simulink subsystem "FORCESANDTORQUES"  (R2025b)
settings: Solver=VariableStepAuto  StartTime=0.0  StopTime=10.0  RelTol=1e-3
model mask{refSurf=0, dc=0}
  mask prompts: refSurf "Reference aerodynamic surface [m2]"; dc "Drag coefficient [-]"
libraries: sharedutil x1, aerolibutil x1
settings Model: Creator=antoniohernandez-rodiciomateos  LastModifiedBy=antoniohernandez-rodiciomateos

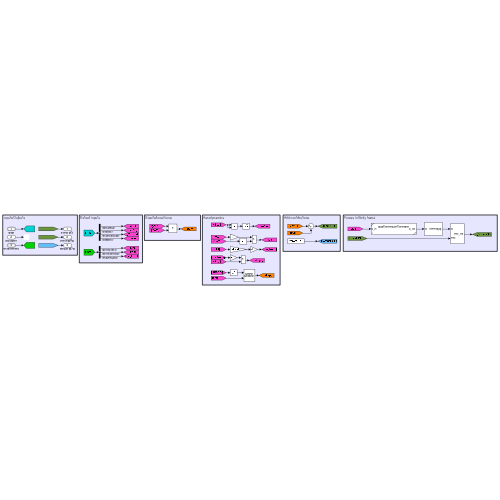
[thumbnail: Simulink's stored preview of the top-level diagram]
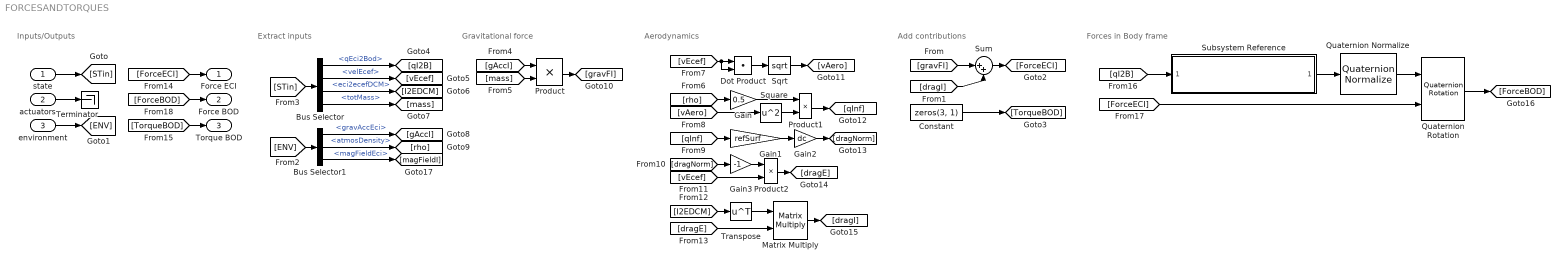
== system FORCESANDTORQUES ==
  note: Inputs/Outputs
  note: Extract inputs
  note: Gravitational force
  note: Aerodynamics
  note: Add contributions
  note: Forces in Body frame
  state : Inport  OutDataTypeStr=Bus: state_bus
  actuators : Inport  Port=2
  environment : Inport  Port=3  OutDataTypeStr=Bus: environment_bus
  Bus Selector : BusSelector  OutputSignals=qEci2Bod,velEcef,eci2ecefDCM,totMass
  Bus Selector1 : BusSelector  OutputSignals=gravAccEci,atmosDensity,magFieldEci
  Constant : Constant  Value=zeros(3, 1)
  Dot Product : DotProduct  OutDataTypeStr=Inherit: Inherit via internal rule
  Gain : Gain  Gain=0.5
  Gain1 : Gain  Gain=refSurf
  Gain2 : Gain  Gain=dc
  Gain3 : Gain  Gain=-1
  Matrix Multiply : Product  Multiplication=Matrix(*)
  Product : Product
  Product1 : Product
  Product2 : Product
  Quaternion Normalize : sharedutil/Quaternion Normalize  aMode=aMode
  Quaternion Rotation : aerolibutil/Quaternion Rotation
  Sqrt : Sqrt
  Square : Math  Operator=square
  Subsystem Reference : Subsystem  ReferencedSubsystem=quatConventionConverter  conversion=q4 to q0
  Sum : Sum  Inputs=|++
  Terminator : Terminator
  Transpose : Math  Operator=transpose
  Force ECI : Outport  OutDataTypeStr=double  PortDimensions=[3 1]
  Force BOD : Outport  Port=2  OutDataTypeStr=double  PortDimensions=[3 1]
  Torque BOD : Outport  Port=3  OutDataTypeStr=double  PortDimensions=[3 1]
  wires:
  actuators/1 -> Terminator/1
  state/1 -> [STin]
  environment/1 -> [ENV]
  [ForceECI] -> Force ECI/1
  [STin] -> Bus Selector/1
  Bus Selector/1 -> [qI2B]  "<qEci2Bod>"
  Bus Selector/2 -> [vEcef]  "<velEcef>"
  Bus Selector/3 -> [I2EDCM]  "<eci2ecefDCM>"
  Bus Selector/4 -> [mass]  "<totMass>"
  [ENV] -> Bus Selector1/1
  Bus Selector1/1 -> [gAccI]  "<gravAccEci>"
  Bus Selector1/2 -> [rho]  "<atmosDensity>"
  [gAccI] -> Product/1
  [mass] -> Product/2
  Product/1 -> [gravFI]
  [vEcef] -> Dot Product/2, Dot Product/1
  Dot Product/1 -> Sqrt/1
  Sqrt/1 -> [vAero]
  [rho] -> Gain/1
  [vAero] -> Square/1
  Gain/1 -> Product1/1
  Square/1 -> Product1/2
  Product1/1 -> [qInf]
  [qInf] -> Gain1/1
  Gain1/1 -> Gain2/1
  Gain2/1 -> [dragNorm]
  [dragNorm] -> Gain3/1
  Gain3/1 -> Product2/1
  [vEcef] -> Product2/2
  Product2/1 -> [dragE]
  [I2EDCM] -> Transpose/1
  Transpose/1 -> Matrix Multiply/1
  [dragE] -> Matrix Multiply/2
  Matrix Multiply/1 -> [dragI]
  [TorqueBOD] -> Torque BOD/1
  [gravFI] -> Sum/1
  [dragI] -> Sum/2
  Sum/1 -> [ForceECI]
  Constant/1 -> [TorqueBOD]
  [qI2B] -> Subsystem Reference/1
  Subsystem Reference/1 -> Quaternion Normalize/1
  Quaternion Normalize/1 -> Quaternion Rotation/1
  [ForceECI] -> Quaternion Rotation/2
  Quaternion Rotation/1 -> [ForceBOD]
  [ForceBOD] -> Force BOD/1
  Bus Selector1/3 -> [magFieldI]  "<magFieldEci>"
